simulink library "AD_Stepper_motor_lib"  (Simulink 7.4)
settings: Solver=ode45  SolverMode=SingleTasking  StartTime=0.0  StopTime=10.0  RelTol=1e-3
undefined symbols (not defined in the file or in its folder): Tmax, Ts
libraries: simulink x2
settings Model: Creator=fw  LastModifiedBy=fw

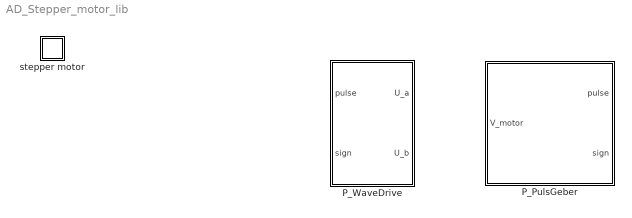
== system AD_Stepper_motor_lib ==
  P_PulsGeber : Subsystem  TreatAsAtomicUnit=on  SystemSampleTime=Ts
  P_WaveDrive : Subsystem  TreatAsAtomicUnit=on  SystemSampleTime=Ts
  stepper motor : Subsystem

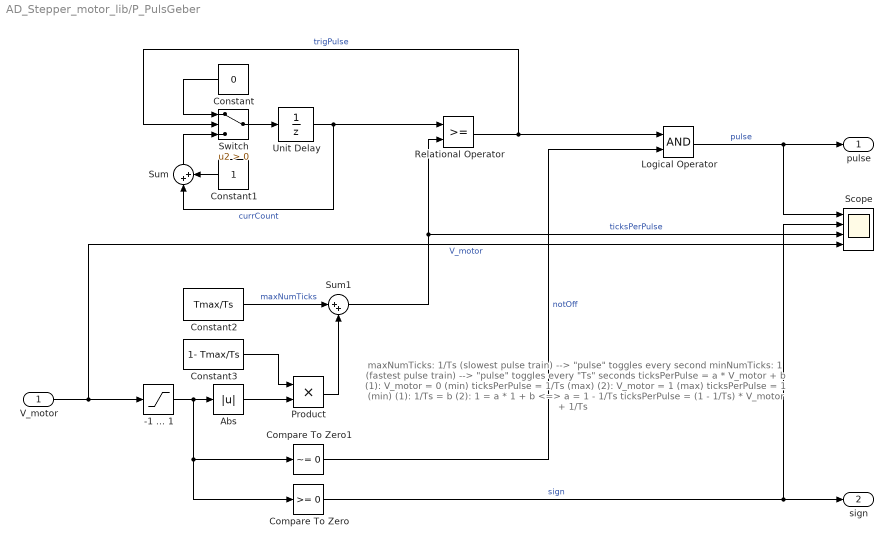
== system AD_Stepper_motor_lib/P_PulsGeber ==
  note: maxNumTicks:  1/Ts   (slowest pulse train)
      | --> "pulse" toggles every second
      | minNumTicks: 1  (fastest pulse train)
      | --> "pulse" toggles every "Ts" seconds
      |
      | ticksPerPulse = a * V_motor + b
      |
      | (1):  V_motor = 0 (min)
      |        ticksPerPulse = 1/Ts (max)
      | (2):  V_motor = 1 (max)
      |        ticksPerPulse = 1 (min)
      |
      | (1):  1/Ts = b
      | (2):  1 = a * 1 + b   <=>   a = 1 - 1/Ts
      |
      | ticksPerPulse = (1 - 1/Ts) * V_motor + 1/Ts
  V_motor : Inport  OutDataType=sfix(16)  OutScaling=2^0
  -1 ... 1 : Saturate  UpperLimit=1  LowerLimit=-1  OutDataType=fixdt(1, 16)  OutScaling=2^0
  Abs : Abs
  Compare To Zero : simulink/Logic and Bit Operations/Compare To Zero  SystemSampleTime=-1  relop=>=  LogicOutDataTypeMode=boolean  ZeroCross=off
  Compare To Zero1 : simulink/Logic and Bit Operations/Compare To Zero  SystemSampleTime=-1  relop=~=  LogicOutDataTypeMode=boolean  ZeroCross=off
  Constant : Constant  Value=0  OutDataType=sfix(16)  OutScaling=2^0
  Constant1 : Constant  OutDataType=sfix(16)  OutScaling=2^0
  Constant2 : Constant  Value=Tmax/Ts  OutDataType=sfix(16)  OutScaling=2^0
  Constant3 : Constant  Value=1- Tmax/Ts  OutDataType=sfix(16)  OutScaling=2^0
  Logical Operator : Logic  AllPortsSameDT=off  OutDataTypeMode=boolean  LogicDataType=fixdt(0, 8)  OutDataTypeStr=boolean
  Product : Product  OutDataType=sfix(16)  OutScaling=2^0  RndMeth=Zero
  Relational Operator : RelationalOperator  LogicOutDataTypeMode=boolean  OutDataTypeStr=boolean
  Scope : Scope  NumInputPorts=4
      settings: TimeRange=10  YMin=-1~-1~0~-1.5  YMax=2~2~60~1.5
  Sum : Sum  Inputs=|++  OutDataType=sfix(16)  OutScaling=2^0
  Sum1 : Sum  Inputs=|++  OutDataType=sfix(16)  OutScaling=2^0
  Switch : Switch  Criteria=u2 > Threshold
  Unit Delay : UnitDelay  SampleTime=Ts
  pulse : Outport  OutDataType=sfix(16)  OutScaling=2^0
  sign : Outport  Port=2  OutDataType=sfix(16)  OutScaling=2^0
  wires:
  Constant2/1 -> Sum1/1  "maxNumTicks"
  Product/1 -> Sum1/2
  Compare To Zero/1 -> sign/1, Scope/2  "sign"
  Constant/1 -> Switch/1
  Relational Operator/1 -> Switch/2, Logical Operator/1  "trigPulse"
  Unit Delay/1 -> Relational Operator/1, Sum/1  "currCount"
  Switch/1 -> Unit Delay/1
  Sum/1 -> Switch/3
  Constant1/1 -> Sum/2
  Abs/1 -> Product/2
  Constant3/1 -> Product/1
  -1 ... 1/1 -> Abs/1, Compare To Zero/1, Compare To Zero1/1
  Sum1/1 -> Relational Operator/2, Scope/3  "ticksPerPulse"
  V_motor/1 -> -1 ... 1/1, Scope/4  "V_motor"
  Logical Operator/1 -> pulse/1, Scope/1  "pulse"
  Compare To Zero1/1 -> Logical Operator/2  "notOff"

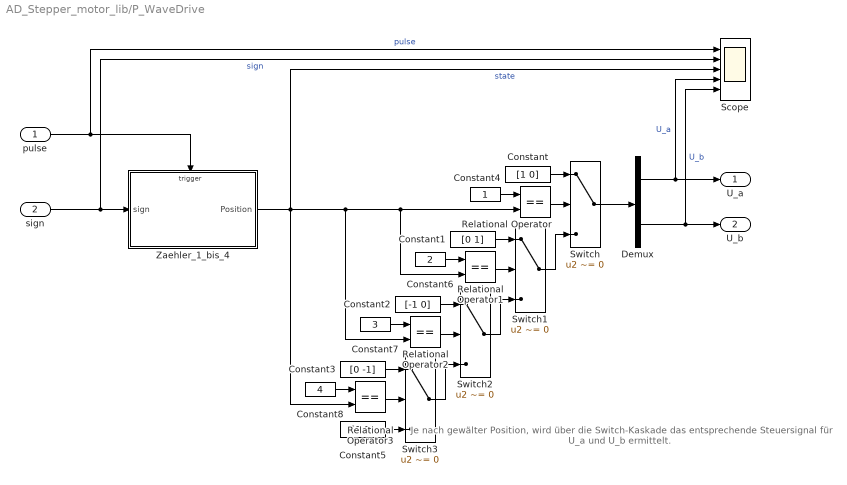
== system AD_Stepper_motor_lib/P_WaveDrive ==
  note: Je nach gewälter Position, wird über die Switch-Kaskade
      | das entsprechende Steuersignal für U_a und U_b
      | ermittelt.
  pulse : Inport  OutDataType=sfix(16)  OutScaling=2^0
  sign : Inport  Port=2  OutDataType=sfix(16)  OutScaling=2^0
  Constant : Constant  Value=[1 0]  OutDataType=sfix(16)  OutScaling=2^0
  Constant1 : Constant  Value=[0 1]  OutDataType=sfix(16)  OutScaling=2^0
  Constant2 : Constant  Value=[-1 0]  OutDataType=sfix(16)  OutScaling=2^0
  Constant3 : Constant  Value=[0 -1]  OutDataType=sfix(16)  OutScaling=2^0
  Constant4 : Constant  OutDataType=sfix(16)  OutScaling=2^0
  Constant5 : Constant  Value=[0 0]  OutDataType=sfix(16)  OutScaling=2^0
  Constant6 : Constant  Value=2  OutDataType=sfix(16)  OutScaling=2^0
  Constant7 : Constant  Value=3  OutDataType=sfix(16)  OutScaling=2^0
  Constant8 : Constant  Value=4  OutDataType=sfix(16)  OutScaling=2^0
  Demux : Demux  Outputs=2
  Relational Operator{,1..3} (4 alike) : RelationalOperator  Operator===  LogicOutDataTypeMode=boolean  OutDataTypeStr=boolean
  Scope : Scope  NumInputPorts=5
      settings: TimeRange=10  YMin=-1~-1~-0~-2~-2  YMax=2~2~5~2~2  SaveName=ScopeData2
  Switch{,1..3} (4 alike) : Switch  Criteria=u2 ~= 0
  Zaehler_1_bis_4 : Subsystem  TreatAsAtomicUnit=on
  U_a : Outport  OutDataType=sfix(16)  OutScaling=2^0
  U_b : Outport  Port=2  OutDataType=sfix(16)  OutScaling=2^0
  wires:
  Demux/2 -> U_b/1, Scope/5  "U_b"
  Demux/1 -> U_a/1, Scope/4  "U_a"
  Zaehler_1_bis_4/1(Position) -> Scope/3, Relational Operator3/2, Relational Operator2/2, Relational Operator1/2, Relational Operator/2  "state"
  sign/1 -> Zaehler_1_bis_4/1(sign), Scope/2  "sign"
  pulse/1 -> Zaehler_1_bis_4/Trigger, Scope/1  "pulse"
  Switch/1 -> Demux/1
  Constant5/1 -> Switch3/3
  Switch3/1 -> Switch2/3
  Relational Operator3/1 -> Switch3/2
  Constant3/1 -> Switch3/1
  Constant8/1 -> Relational Operator3/1
  Switch2/1 -> Switch1/3
  Relational Operator2/1 -> Switch2/2
  Constant2/1 -> Switch2/1
  Constant7/1 -> Relational Operator2/1
  Switch1/1 -> Switch/3
  Relational Operator1/1 -> Switch1/2
  Constant1/1 -> Switch1/1
  Constant6/1 -> Relational Operator1/1
  Relational Operator/1 -> Switch/2
  Constant/1 -> Switch/1
  Constant4/1 -> Relational Operator/1

== system AD_Stepper_motor_lib/stepper motor ==

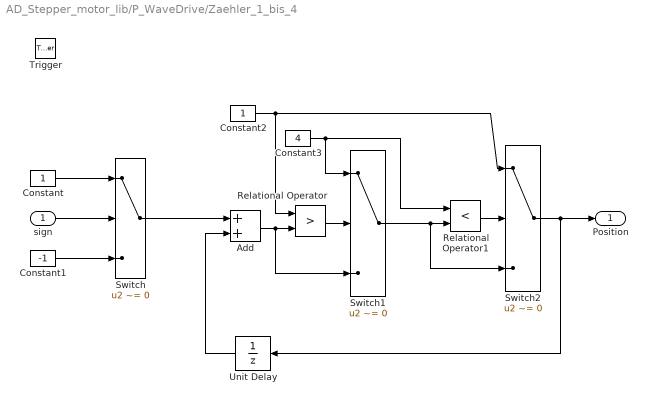
== system AD_Stepper_motor_lib/P_WaveDrive/Zaehler_1_bis_4 ==
  sign : Inport  OutDataType=sfix(16)  OutScaling=2^0
  Trigger : TriggerPort
  Add : Sum  OutDataType=sfix(16)  OutScaling=2^-10
  Constant : Constant  OutDataType=sfix(16)  OutScaling=2^0
  Constant1 : Constant  Value=-1  OutDataType=sfix(16)  OutScaling=2^0
  Constant2 : Constant  OutDataType=sfix(16)  OutScaling=2^0
  Constant3 : Constant  Value=4  OutDataType=sfix(16)  OutScaling=2^0
  Relational Operator : RelationalOperator  Operator=>  LogicOutDataTypeMode=boolean  OutDataTypeStr=boolean
  Relational Operator1 : RelationalOperator  Operator=<  LogicOutDataTypeMode=boolean  OutDataTypeStr=boolean
  Switch : Switch  Criteria=u2 ~= 0
  Switch1 : Switch  Criteria=u2 ~= 0
  Switch2 : Switch  Criteria=u2 ~= 0
  Unit Delay : UnitDelay  X0=1  SampleTime=-1
  Position : Outport  OutDataType=sfix(16)  OutScaling=2^0
  wires:
  Switch2/1 -> Unit Delay/1, Position/1
  Relational Operator1/1 -> Switch2/2
  Switch1/1 -> Switch2/3, Relational Operator1/2
  Relational Operator/1 -> Switch1/2
  Constant3/1 -> Relational Operator1/1, Switch1/1
  Add/1 -> Switch1/3, Relational Operator/2
  Constant2/1 -> Switch2/1, Relational Operator/1
  Unit Delay/1 -> Add/2
  Switch/1 -> Add/1
  Constant1/1 -> Switch/3
  sign/1 -> Switch/2
  Constant/1 -> Switch/1
